simulink model "ElectricalModel_estimation_CRate"  (R2020b)
settings: Solver=FixedStepDiscrete  StartTime=0.0  StopTime=runTime  FixedStep=stepSize
values from neighbouring files (symbols this model uses):
  init_I1 = simout_init.I1(end)    [CRate_process.m]
  init_I2 = simout_init.I2(end)    [CRate_process.m]
  init_I3 = simout_init.I3(end)    [CRate_process.m]
  init_SOC = simout_init.SOC(end)    [CRate_process.m]
  OCV_current = param_current.OCV_opt    [CRate_process.m]
  OCV_prev = param_prev.OCV_opt    [CRate_process.m]
  R0_current = param_current.R0_opt    [CRate_process.m]
  R0_prev = param_prev.R0_opt    [CRate_process.m]
  R1_current = param_current.R1_opt    [CRate_process.m]
  R1_prev = param_prev.R1_opt    [CRate_process.m]
  R2_current = param_current.R2_opt    [CRate_process.m]
  R2_prev = param_prev.R2_opt    [CRate_process.m]
  R3_current = param_current.R3_opt    [CRate_process.m]
  R3_prev = param_prev.R3_opt    [CRate_process.m]
  SOC_current = param_current.SOC    [CRate_process.m]
  SOC_prev = param_prev.SOC    [CRate_process.m]
  tau1_current = param_current.tau1_opt    [CRate_process.m]
  tau1_prev = param_prev.tau1_opt    [CRate_process.m]
  tau2_current = param_current.tau2_opt    [CRate_process.m]
  tau2_prev = param_prev.tau2_opt    [CRate_process.m]
  tau3_current = param_current.tau3_opt    [CRate_process.m]
  tau3_prev = param_prev.tau3_opt    [CRate_process.m]
undefined symbols (not defined in the file or in its folder): OCV, Q, SOC
settings Model: OrderedModelArguments=off  Creator=Wenlin  LastModifiedBy=Wenlin
settings DataIOCC: OutputOption=AdditionalOutputTimes  OutputTimes=SDO_OutputTimes  ReturnWorkspaceOutputsName=SDOSimTest_Log
settings DebuggingCC: UnderSpecifiedDimensionMsg=warning

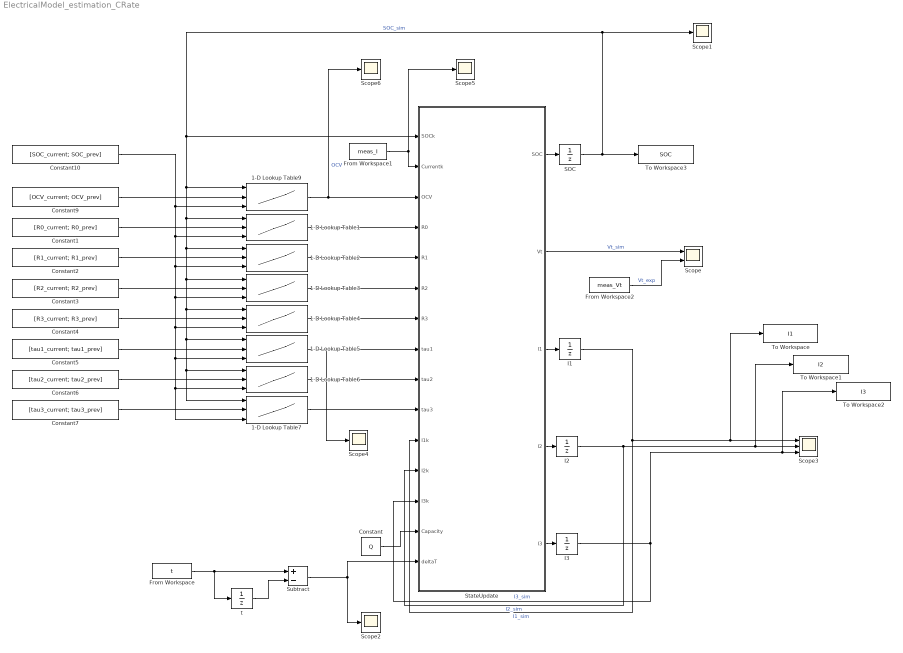
== system ElectricalModel_estimation_CRate ==
  1-D Lookup Table{1..7,9} (8 alike) : Lookup_n-D  NumberOfTableDimensions=1  BreakpointsForDimension1Source=Input port  BreakpointsForDimension1=SOC  TableSource=Input port  Table=OCV  InternalRulePriority=Speed  RndMeth=Simplest  InputSameDT=on
      settings: InputPortMap=u0,p221,p5
  Constant : Constant  Value=Q
  Constant1 : Constant  Value=[R0_current; R0_prev]
  Constant10 : Constant  Value=[SOC_current; SOC_prev]
  Constant2 : Constant  Value=[R1_current; R1_prev]
  Constant3 : Constant  Value=[R2_current; R2_prev]
  Constant4 : Constant  Value=[R3_current; R3_prev]
  Constant5 : Constant  Value=[tau1_current; tau1_prev]
  Constant6 : Constant  Value=[tau2_current; tau2_prev]
  Constant7 : Constant  Value=[tau3_current; tau3_prev]
  Constant9 : Constant  Value=[OCV_current; OCV_prev]
  From Workspace : FromWorkspace  VariableName=t  OutputAfterFinalValue=Setting to zero
  From Workspace1 : FromWorkspace  VariableName=meas_I
  From Workspace2 : FromWorkspace  VariableName=meas_Vt
  I1 : UnitDelay  InitialCondition=init_I1  SampleTime=-1  HasFrameUpgradeWarning=on
  I2 : UnitDelay  InitialCondition=init_I2  SampleTime=-1  HasFrameUpgradeWarning=on
  I3 : UnitDelay  InitialCondition=init_I3  SampleTime=-1  HasFrameUpgradeWarning=on
  SOC : UnitDelay  InitialCondition=init_SOC  SampleTime=-1  HasFrameUpgradeWarning=on
  Scope : Scope  NumInputPorts=2
  Scope{1..2,4..6} (5 alike) : Scope
  Scope3 : Scope  NumInputPorts=3
  StateUpdate : MATLAB Function  TreatAsAtomicUnit=on
  Subtract : Sum  Inputs=+-
  To Workspace : ToWorkspace  VariableName=I1  SampleTime=-1
  To Workspace1 : ToWorkspace  VariableName=I2  SampleTime=-1
  To Workspace2 : ToWorkspace  VariableName=I3  SampleTime=-1
  To Workspace3 : ToWorkspace  VariableName=SOC  SampleTime=-1
  t : UnitDelay  SampleTime=-1  HasFrameUpgradeWarning=on
  wires:
  Constant6/1 -> 1-D Lookup Table6/2
  StateUpdate/1(SOC) -> SOC/1
  Constant7/1 -> 1-D Lookup Table7/2
  I2/1 -> To Workspace1/1, Scope3/2, StateUpdate/12(I2k)  "I2_sim"
  Constant4/1 -> 1-D Lookup Table4/2
  StateUpdate/4(I2) -> I2/1
  Constant5/1 -> 1-D Lookup Table5/2
  1-D Lookup Table6/1 -> StateUpdate/9(tau2)
  Constant/1 -> StateUpdate/14(Capacity)
  1-D Lookup Table1/1 -> StateUpdate/4(R0)
  Constant2/1 -> 1-D Lookup Table2/2
  1-D Lookup Table2/1 -> StateUpdate/5(R1)
  From Workspace/1 -> t/1, Subtract/1
  Constant1/1 -> 1-D Lookup Table1/2
  I1/1 -> StateUpdate/11(I1k), To Workspace/1, Scope3/1  "I1_sim"
  1-D Lookup Table4/1 -> StateUpdate/7(R3)
  Constant10/1 -> 1-D Lookup Table9/3, 1-D Lookup Table7/3, 1-D Lookup Table6/3, 1-D Lookup Table5/3, 1-D Lookup Table4/3, 1-D Lookup Table3/3, 1-D Lookup Table2/3, 1-D Lookup Table1/3
  StateUpdate/2(Vt) -> Scope/1  "Vt_sim"
  Subtract/1 -> Scope2/1, StateUpdate/15(deltaT)
  1-D Lookup Table9/1 -> Scope6/1, StateUpdate/3(OCV)  "OCV"
  StateUpdate/3(I1) -> I1/1
  t/1 -> Subtract/2
  From Workspace1/1 -> Scope5/1, StateUpdate/2(Currentk)
  SOC/1 -> To Workspace3/1, Scope1/1, 1-D Lookup Table1/1, 1-D Lookup Table7/1, 1-D Lookup Table6/1, 1-D Lookup Table5/1, 1-D Lookup Table4/1, 1-D Lookup Table3/1, 1-D Lookup Table2/1, 1-D Lookup Table9/1, StateUpdate/1(SOCk)  "SOC_sim"
  StateUpdate/5(I3) -> I3/1
  1-D Lookup Table3/1 -> StateUpdate/6(R2)
  Constant3/1 -> 1-D Lookup Table3/2
  1-D Lookup Table5/1 -> Scope4/1, StateUpdate/8(tau1)
  1-D Lookup Table7/1 -> StateUpdate/10(tau3)
  I3/1 -> To Workspace2/1, Scope3/3, StateUpdate/13(I3k)  "I3_sim"
  Constant9/1 -> 1-D Lookup Table9/2
  From Workspace2/1 -> Scope/2  "Vt_exp"

== matlab function ElectricalModel_estimation_CRate/StateUpdate ==
  data: SOC output; SOCk input; Currentk input; OCV input; R0 input; R1 input; R2 input; R3 input; tau1 input; tau2 input; tau3 input; I1k input; I2k input; I3k input; Capacity input; deltaT input; Vt output; I1 output; I2 output; I3 output
function [SOC, Vt, I1, I2, I3] = StateUpdate(SOCk, Currentk, OCV, R0, R1, R2, R3, tau1, tau2, tau3, I1k, I2k, I3k, Capacity, deltaT)

    Q = Capacity*3600;
%     if tau1 <0
%         A = 0;
%     end
    % Calculate currents
    I1 =  ( 1 - exp(-deltaT/tau1) ) * Currentk + exp(-deltaT/tau1) * I1k;
    I2 =  ( 1 - exp(-deltaT/tau2) ) * Currentk + exp(-deltaT/tau2) * I2k;
    I3 =  ( 1 - exp(-deltaT/tau3) ) * Currentk + exp(-deltaT/tau3) * I3k;
%     if abs(I1) >280
%         A = 0;
%     end
    % Update voltage & SOC
    Vt   = OCV + (R0*Currentk) + R1*I1 + R2*I2 + R3*I3;
%     if Vt<2.5
%        A  = 0; 
%     end
    SOC  = SOCk + (deltaT/Q) * Currentk;

end
